simulink model "directed_event"  (R2020a)
settings: Solver=VariableStepAuto  StartTime=0.0  StopTime=0.1  RelTol=1e-3
settings Model: Creator=86188  LastModifiedBy=bzhan
settings DataIOCC: ReturnWorkspaceOutputs=off
settings DebuggingCC: ArithmeticOperatorsInVariantConditions=warning
settings SFSimCC: SimUseLocalCustomCode=off  CustomCodeUndefinedFunction=UseInterfaceOnly
settings RTWCC: RTWUseLocalCustomCode=off

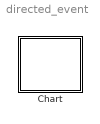
== system directed_event ==
  Chart : Stateflow chart  TreatAsAtomicUnit=on

== stateflow chart directed_event/Chart ==
  settings: updateMethod=DISCRETE  sampleTime=0.1  executeAtInitialization=1
  state AM
    state A [parallel]
      settings: executionOrder=1
      state A1
        en: f("en_A1")
        ex: f("ex_A1")
      state A2
        en: f("en_A2")
        ex: f("ex_A2")
      (default) -> A1
      A1 -> A2 : [data==1]{B.E_one}
      A2 -> A1 : E_two
    state B [parallel]
      settings: executionOrder=2
      state B1
        en: f("en_B1")
        ex: f("ex_B1")
      state B2
        en: f("en_B2")
        ex: f("ex_B2")
      (default) -> B1
      B1 -> B2 : E_one{C.E_one}
      B2 -> B1 : E_two{A.E_two}
    state C [parallel]
      settings: executionOrder=3
      state C1
        en: f("en_C1")
        ex: f("ex_C1")
      state C2
        en: f("en_C2")
        ex: f("ex_C2")
      (default) -> C1
      C1 -> C2 : E_one
      C2 -> C1 : [data==1]{B.E_two}
  (default) -> AM : {data = 1}
  data: s function_input; data local double =1
  events: E_two local FUNCTION_CALL_EVENT; E_one local FUNCTION_CALL_EVENT; E_two local FUNCTION_CALL_EVENT; E_one local FUNCTION_CALL_EVENT
  function f(s):
    | function f(s)
    |   fprintf(s+"\n");
